simulink model "PHREG"  (R2025a)
settings: Solver=FixedStepDiscrete  StartTime=0.0  StopTime=500  FixedStep=0.2  RelTol=1e-3
libraries: slpidlib x1
settings Model: Creator=HP  LastModifiedBy=HP

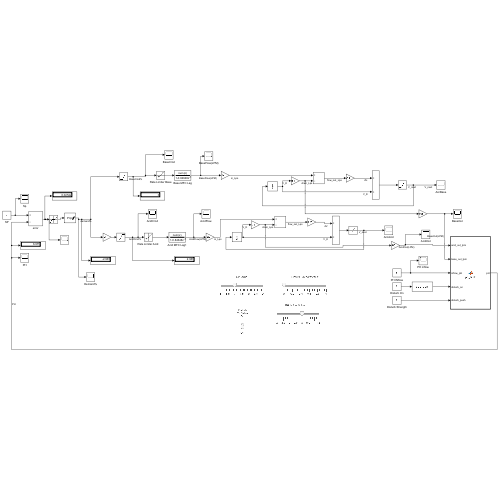
[thumbnail: Simulink's stored preview of the top-level diagram]
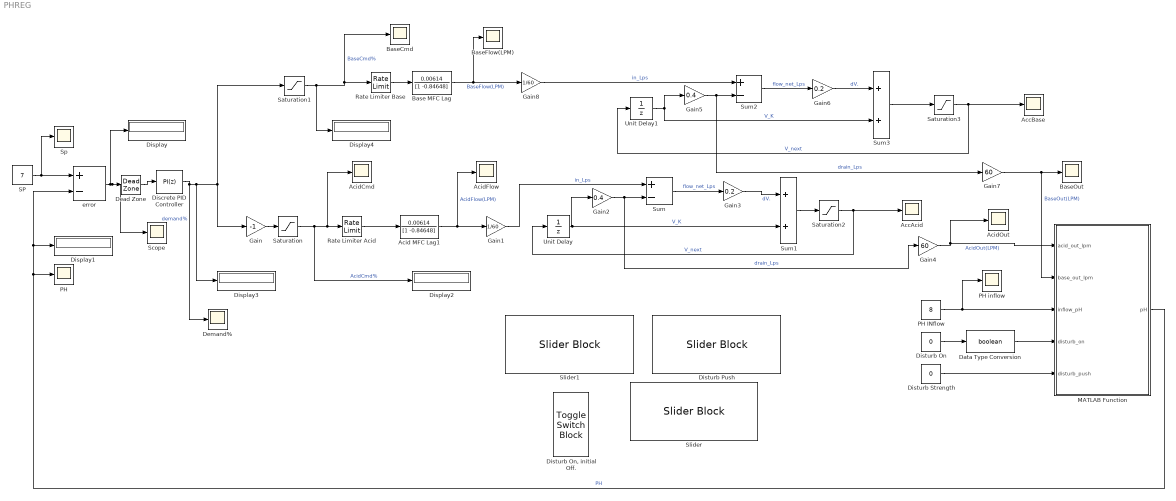
== system PHREG ==
  AccAcid : Scope
      settings: ActiveDisplayYMinimum=-1.9227261584179611  ActiveDisplayYMaximum=1.3449815656648016  DataLoggingVariableName=ScopeData10
  AccBase : Scope
      settings: ActiveDisplayYMinimum=-1  ActiveDisplayYMaximum=1  DataLoggingVariableName=ScopeData9
  Acid MFC Lag1 : DiscreteFilter  Numerator=0.00614  Denominator=[1 -0.84648]
  AcidCmd : Scope
      settings: ActiveDisplayYMinimum=-6.1712758270621428  ActiveDisplayYMaximum=45.945096040862666  DataLoggingVariableName=ScopeData4
  AcidFlow : Scope
      settings: ActiveDisplayYMinimum=-2.3952148191729949  ActiveDisplayYMaximum=2.3919204627810644  DataLoggingVariableName=ScopeData6
  AcidOut : Scope
      settings: ActiveDisplayYMinimum=-0.033965860536458718  ActiveDisplayYMaximum=0.30569274482812853  DataLoggingVariableName=ScopeData8
  Base MFC Lag : DiscreteFilter  Numerator=0.00614  Denominator=[1 -0.84648]
  BaseCmd : Scope
      settings: ActiveDisplayYMinimum=-1  ActiveDisplayYMaximum=1  DataLoggingVariableName=ScopeData2
  BaseFlow(LPM) : Scope
      settings: ActiveDisplayYMinimum=-8.4461988069918021  ActiveDisplayYMaximum=5.8060315030331537  DataLoggingVariableName=ScopeData5
  BaseOut : Scope
      settings: ActiveDisplayYMinimum=-0.22107048052200748  ActiveDisplayYMaximum=0.27462947756705169  DataLoggingVariableName=ScopeData7
  Data Type Conversion : DataTypeConversion  OutDataTypeStr=boolean  SaturateOnIntegerOverflow=off  RndMeth=Floor
  Dead Zone : DeadZone  LowerValue=-0.02  UpperValue=0.02
  Demand% : Scope
      settings: ActiveDisplayYMinimum=-41.78406737615876  ActiveDisplayYMaximum=2.46489637512875
  Discrete PID Controller : slpidlib/PID Controller  Controller=PI  Form=Parallel  TimeDomain=Discrete-time  UseExternalTs=off  SampleTime=0.2  IntegratorMethod=Forward Euler  FilterMethod=Forward Euler  ControllerParametersSource=internal  P=3.2  I=0.16  UseKiTs=off  D=0  UseExternalDerivativeSource=off  N=100  UseFilter=on  TunerSelectOption=Transfer Function Based (PID Tuner App)  InitialConditionSource=internal  InitialConditionForIntegrator=0  InitialConditionForFilter=0  DifferentiatorICPrevScaledInput=0  ExternalReset=none  TrackingMode=off  Kt=1  LimitOutput=on  SatLimitsSource=internal  UpperSaturationLimit=40  LowerSaturationLimit=-40  LinearizeAsGain=off  AntiWindupMode=back-calculation  Kb=1  LimitIntegrator=on  UpperIntegratorSaturationLimit=40  LowerIntegratorSaturationLimit=-40  POutMin=[]  POutMax=[]  IOutMin=[]  IOutMax=[]  DOutMin=[]  DOutMax=[]  NOutMin=[]  NOutMax=[]  SumOutMin=[]  SumOutMax=[]  SaturationOutMin=[]  SaturationOutMax=[]  PParamMin=[]  PParamMax=[]  IParamMin=[]  IParamMax=[]  DParamMin=[]  DParamMax=[]  NParamMin=[]  NParamMax=[]  KbParamMin=[]  KbParamMax=[]  KtParamMin=[]  KtParamMax=[]  KbOutMin=[]  KbOutMax=[]  KtOutMin=[]  KtOutMax=[]  IntegratorOutMin=[]  IntegratorOutMax=[]  FilterOutMin=[]  FilterOutMax=[]  SumI1OutMin=[]  SumI1OutMax=[]  SumI2OutMin=[]  SumI2OutMax=[]  SumI3OutMin=[]  SumI3OutMax=[]  SumI4OutMin=[]  SumI4OutMax=[]  SumDOutMin=[]  SumDOutMax=[]  DifferentiatorOutMin=[]  DifferentiatorOutMax=[]  FilterDiffOutCoefMin=[]  FilterDiffOutCoefMax=[]  ReciprocalOutMin=[]  ReciprocalOutMax=[]  SumDenOutMin=[]  SumDenOutMax=[]  SumNumOutMin=[]  SumNumOutMax=[]  DivideOutMin=[]  DivideOutMax=[]  UdiffTsProdOutMin=[]  UdiffTsProdOutMax=[]  NTsProdOutMin=[]  NTsProdOutMax=[]  UintegralTsProdOutMin=[]  UintegralTsProdOutMax=[]  UngainTsProdOutMin=[]  UngainTsProdOutMax=[]  ClampingZeroOutDataTypeStr=Inherit: Inherit via back propagation  ClampingZeroOutMin=[]  ClampingZeroOutMax=[]  FilterDenConstantOutDataTypeStr=Inherit: Inherit via back propagation  FilterDenConstantOutMin=[]  FilterDenConstantOutMax=[]  PCopyOutDataTypeStr=Inherit: Inherit via back propagation  PCopyOutMin=[]  PCopyOutMax=[]  NCopyOutDataTypeStr=Inherit: Inherit via back propagation  NCopyOutMin=[]  NCopyOutMax=[]  IntegratorContinuousStateAttributes=''  IntegratorStateMustResolveToSignalObject=off  IntegratorRTWStateStorageClass=Auto  FilterContinuousStateAttributes=''  FilterStateMustResolveToSignalObject=off  FilterRTWStateStorageClass=Auto  ParallelPVariant=InternalParameters  IdealPVariant=Disabled  IVariant=InternalParameters  DVariant=Disabled  IntegratorVariant=Discrete  SatVariant=Enabled  AWVariant=BackCalculation  PCopyVariant=Disabled  TRVariant=Disabled  FdbkBlocksVariant=Forward  IdealPFdbkVariant=Disabled  SatFdbkVariant=Disabled  DerivativeFilterVariant=Disabled  NVariant=Disabled  NCopyVariant=Disabled_SignalSpec  FilterICVariant=Disabled  IntegratorICVariant=InternalICs  ExternalResetVariant=Disabled  TRSumVariant=Passthrough  SumFdbkVariant=Disabled  SumVariant=Sum_PI  TsampFilterVariant=InternalTs  TsampNgainVariant=Passthrough  TsampIntegralVariant=Disabled_SignalSpec  ExternalSaturationOutDataTypeStr=Inherit: Same as second input  DerivativeSourceVariant=Disabled  PreIntVariant=InternalPreInt
      settings: LibrarySourceBlock=simulink/Discrete/Discrete PID Controller
  Display{,1..4} (5 alike) : Display
  Disturb On : Constant  Value=0
  "Disturb On, initial Off." : ToggleSwitchBlock
  Disturb Push : SliderBlock  ScaleMax=1
  Disturb Strength : Constant  Value=0
  Gain : Gain  Gain=-1
  Gain1 : Gain  Gain=1/60
  Gain2 : Gain  Gain=0.4
  Gain3 : Gain  Gain=0.2
  Gain4 : Gain  Gain=60
  Gain5 : Gain  Gain=0.4
  Gain6 : Gain  Gain=0.2
  Gain7 : Gain  Gain=60
  Gain8 : Gain  Gain=1/60
  MATLAB Function : MATLAB Function  TreatAsAtomicUnit=on
  PH : Scope
      settings: ActiveDisplayYMinimum=6.2696102788878925  ActiveDisplayYMaximum=8.2450358391075316  DataLoggingVariableName=ScopeData11
  PH INflow : Constant  Value=8
  PH inflow : Scope
      settings: ActiveDisplayYMinimum=0.78492040541433916  ActiveDisplayYMaximum=1.2141552672288234  DataLoggingVariableName=ScopeData3
  "Rate Limiter Acid " : RateLimiter  RisingSlewLimit=150  FallingSlewLimit=-150  SampleTimeMode=inherited  InitialCondition=0.2
  Rate Limiter Base : RateLimiter  RisingSlewLimit=150  FallingSlewLimit=-150  SampleTimeMode=inherited  InitialCondition=0.2
  SP : Constant  Value=7
  Saturation : Saturate  UpperLimit=100  LowerLimit=0
  Saturation1 : Saturate  UpperLimit=100  LowerLimit=0
  Saturation2 : Saturate  UpperLimit=0.4  LowerLimit=0
  Saturation3 : Saturate  UpperLimit=0.4  LowerLimit=0
  Scope : Scope
      settings: ActiveDisplayYMinimum=-18.619024413520673  ActiveDisplayYMaximum=13.030392632557247
  Slider : SliderBlock  ScaleMin=2  ScaleMax=12
  Slider1 : SliderBlock  ScaleMin=6  ScaleMax=9
  Sp : Scope
      settings: ActiveDisplayYMinimum=5.89341098891389  ActiveDisplayYMaximum=8.1239545480822333  DataLoggingVariableName=ScopeData12
  Sum : Sum  Inputs=+-
  Sum1 : Sum
  Sum2 : Sum  Inputs=+-
  Sum3 : Sum
  Unit Delay : UnitDelay  SampleTime=0.2  HasFrameUpgradeWarning=on
  Unit Delay1 : UnitDelay  SampleTime=0.2  HasFrameUpgradeWarning=on
  error : Sum  Inputs=+-
  wires:
  SP/1 -> Sp/1, error/1
  error/1 -> Display/1, Scope/1, Dead Zone/1
  Dead Zone/1 -> Discrete PID Controller/1
  Discrete PID Controller/1 -> Demand%/1, Display3/1, Gain/1, Saturation1/1  "demand%"
  Gain/1 -> Saturation/1
  Saturation1/1 -> Display4/1, BaseCmd/1, Rate Limiter Base/1  "BaseCmd%"
  Saturation/1 -> Display2/1, AcidCmd/1, "Rate Limiter Acid "/1  "AcidCmd%"
  Acid MFC Lag1/1 -> AcidFlow/1, Gain1/1  "AcidFlow(LPM)"
  Rate Limiter Base/1 -> Base MFC Lag/1
  "Rate Limiter Acid "/1 -> Acid MFC Lag1/1
  Gain1/1 -> Sum/1  "in_Lps"
  Unit Delay/1 -> Gain2/1, Sum1/2  "V_K"
  Gain2/1 -> Gain4/1, Sum/2  "drain_Lps"
  Sum/1 -> Gain3/1  "flow_net_Lps"
  Gain3/1 -> Sum1/1  "dV."
  Sum1/1 -> Saturation2/1
  Saturation2/1 -> Unit Delay/1, AccAcid/1  "V_next"
  Gain4/1 -> MATLAB Function/1(acid_out_lpm), AcidOut/1  "AcidOut(LPM)"
  Unit Delay1/1 -> Sum3/2, Gain5/1  "V_K"
  Base MFC Lag/1 -> BaseFlow(LPM)/1, Gain8/1  "BaseFlow(LPM)"
  Gain6/1 -> Sum3/1  "dV."
  Sum3/1 -> Saturation3/1
  Saturation3/1 -> AccBase/1, Unit Delay1/1  "V_next"
  Gain5/1 -> Gain7/1, Sum2/2  "drain_Lps"
  Sum2/1 -> Gain6/1  "flow_net_Lps"
  Gain7/1 -> MATLAB Function/2(base_out_lpm), BaseOut/1  "BaseOut(LPM)"
  Gain8/1 -> Sum2/1  "in_Lps"
  PH INflow/1 -> PH inflow/1, MATLAB Function/3(inflow_pH)
  Data Type Conversion/1 -> MATLAB Function/4(disturb_on)
  Disturb On/1 -> Data Type Conversion/1
  Disturb Strength/1 -> MATLAB Function/5(disturb_push)
  MATLAB Function/1(pH) -> Display1/1, error/2, PH/1  "PH"

== matlab function PHREG/MATLAB Function ==
  data: acid_out_lpm input; pH output; base_out_lpm input; inflow_pH input; disturb_on input; disturb_push input
function pH = ph_tank(acid_out_lpm, base_out_lpm, inflow_pH, disturb_on, disturb_push)
%#codegen
persistent pH_state
if isempty(pH_state), pH_state = inflow_pH; end

Ts        = 0.2;     % s (match model)
bufferCap = 0.3;     % larger => slower, more buffered
tau_mix   = 25.0;    % s (mixing time constant)

% Nonlinear sensitivity: more sensitive near pH 7
sens = 1.0 / (bufferCap * (1.0 + 10^(pH_state - 7.0)));

% Dosing pushes (scaled)
acid_push = -0.20 * acid_out_lpm * sens;
base_push = +0.20 * base_out_lpm * sens;

% Optional disturbance
disturb = (disturb_on ~= 0) * disturb_push;

% Inflow mixing toward inflow_pH
mix = (inflow_pH - pH_state) / tau_mix;

% Integrate
dpH = (acid_push + base_push + disturb + mix) * Ts;
pH_state = min(12.0, max(2.0, pH_state + dpH));

pH = pH_state;
